simulink model "modelo_SEIRV"  (R2019b)
settings: Solver=VariableStepAuto  StartTime=0.0  StopTime=365  RelTol=1e-3
settings Model: Creator=lucia  LastModifiedBy=lucia

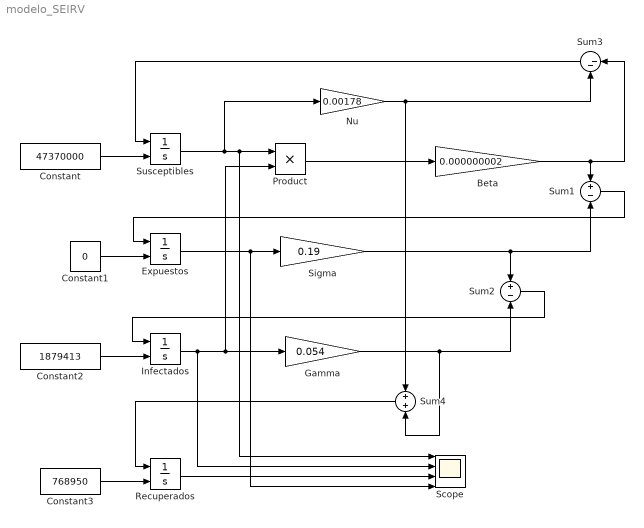
== system modelo_SEIRV ==
  Beta : Gain  Gain=0.000000002
  Constant : Constant  Value=47370000
  Constant1 : Constant  Value=0
  Constant2 : Constant  Value=1879413
  Constant3 : Constant  Value=768950
  Expuestos : Integrator  InitialConditionSource=external
  Gamma : Gain  Gain=0.054
  Infectados : Integrator  InitialConditionSource=external
  Nu : Gain  Gain=0.00178
  Product : Product
  Recuperados : Integrator  InitialConditionSource=external
  Scope : Scope  NumInputPorts=4
  Sigma : Gain  Gain=0.19
  Sum1 : Sum  Inputs=+-
  Sum2 : Sum  Inputs=+-
  Sum3 : Sum  Inputs=|--
  Sum4 : Sum
  Susceptibles : Integrator  InitialConditionSource=external
  wires:
  Sigma/1 -> Sum1/2, Sum2/1
  Recuperados/1 -> Scope/3
  Gamma/1 -> Sum2/2, Sum4/2
  Constant/1 -> Susceptibles/2
  Sum1/1 -> Expuestos/1
  Sum3/1 -> Susceptibles/1
  Sum2/1 -> Infectados/1
  Susceptibles/1 -> Nu/1, Scope/1, Product/1
  Product/1 -> Beta/1
  Constant2/1 -> Infectados/2
  Constant1/1 -> Expuestos/2
  Infectados/1 -> Scope/2, Product/2, Gamma/1
  Beta/1 -> Sum3/1, Sum1/1
  Expuestos/1 -> Scope/4, Sigma/1
  Constant3/1 -> Recuperados/2
  Nu/1 -> Sum3/2, Sum4/1
  Sum4/1 -> Recuperados/1
